simulink model "nonlinPendProvaMia"  (R2018a)
settings: Solver=VariableStepAuto  StartTime=0.0  StopTime=10.0  RelTol=1e-3
values from neighbouring files (symbols this model uses):
  b = 3e-3    (= 0.003)    [DatiPendolo.m]
  g = 9.81    [DatiPendolo.m]
  l = 0.1    [DatiPendolo.m]
  m = 1    [DatiPendolo.m]
settings Model: Creator=bonaventur  LastModifiedBy=bonaventur

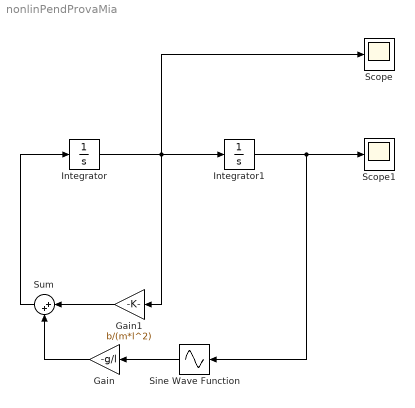
== system nonlinPendProvaMia ==
  Gain : Gain  Gain=-g/l
  Gain1 : Gain  Gain=b/(m*l^2)
  Integrator : Integrator
  Integrator1 : Integrator
  Scope : Scope
  Scope1 : Scope
  Sine Wave Function : Sin  TimeSource=Use external signal  SampleTime=0
  Sum : Sum  Inputs=|++
  wires:
  Integrator/1 -> Gain1/1, Scope/1, Integrator1/1
  Sine Wave Function/1 -> Gain/1
  Gain/1 -> Sum/2
  Gain1/1 -> Sum/1
  Integrator1/1 -> Sine Wave Function/1, Scope1/1
  Sum/1 -> Integrator/1
